simulink model "final_part_2"  (Simulink 8.3)
settings: Solver=ode45  StartTime=0.0  StopTime=60  RelTol=1e-3
undefined symbols (not defined in the file or in its folder): drawMass, P
settings Model: Creator=beard  LastModifiedBy=jhl48
settings DataIOCC: LimitDataPoints=off
settings OptimizationCC: ExpressionDepthLimit=2147483647
settings DebuggingCC: SolverPrmCheckMsg=none  FcnCallInpInsideContextMsg=UseLocalSettings

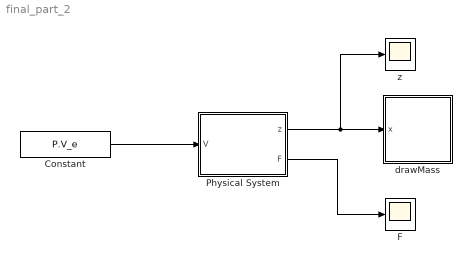
== system final_part_2 ==
  Constant : Constant  Value=P.V_e
  F : Scope
      settings: TimeRange=60  YMin=-4.5  YMax=-2
  Physical System : Subsystem
  drawMass : Subsystem
      mask init:
      | % drawing parameters
      | L = 5;
      | w = 1;
      | theta = 45*pi/180;
      mask Display: image(imread('tv.jpg'))
  z : Scope
      settings: TimeRange=60  YMin=-1  YMax=1
  wires:
  Physical System/1(z) -> drawMass/1(x), z/1
  Constant/1 -> Physical System/1(V)
  Physical System/2(F) -> F/1

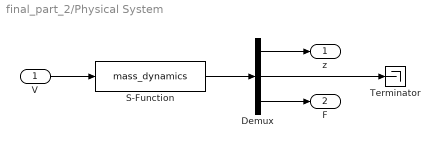
== system final_part_2/Physical System ==
  V : Inport
  Demux : Demux  Outputs=[1;2;1]
  S-Function : S-Function  FunctionName=mass_dynamics  Parameters=P  EnableBusSupport=off
  Terminator : Terminator
  z : Outport
  F : Outport  Port=2
  wires:
  V/1 -> S-Function/1
  S-Function/1 -> Demux/1
  Demux/1 -> z/1
  Demux/3 -> F/1
  Demux/2 -> Terminator/1

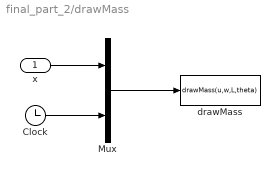
== system final_part_2/drawMass ==
  x : Inport
  Clock : Clock
  Mux : Mux  Inputs=2
  drawMass : MATLABFcn  MATLABFcn=drawMass(u,w,L,theta)  OutputDimensions=0  SampleTime=0.1
  wires:
  Clock/1 -> Mux/2
  x/1 -> Mux/1
  Mux/1 -> drawMass/1
